simulink model "Non_Linear_Disturbance"  (R2024b)
settings: Solver=VariableStepAuto  StartTime=0.0  StopTime=500  RelTol=1e-9
settings Model: Creator=apm3  LastModifiedBy=baley

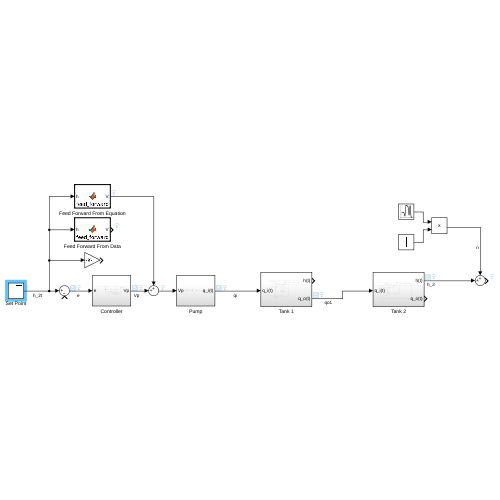
[thumbnail: Simulink's stored preview of the top-level diagram]
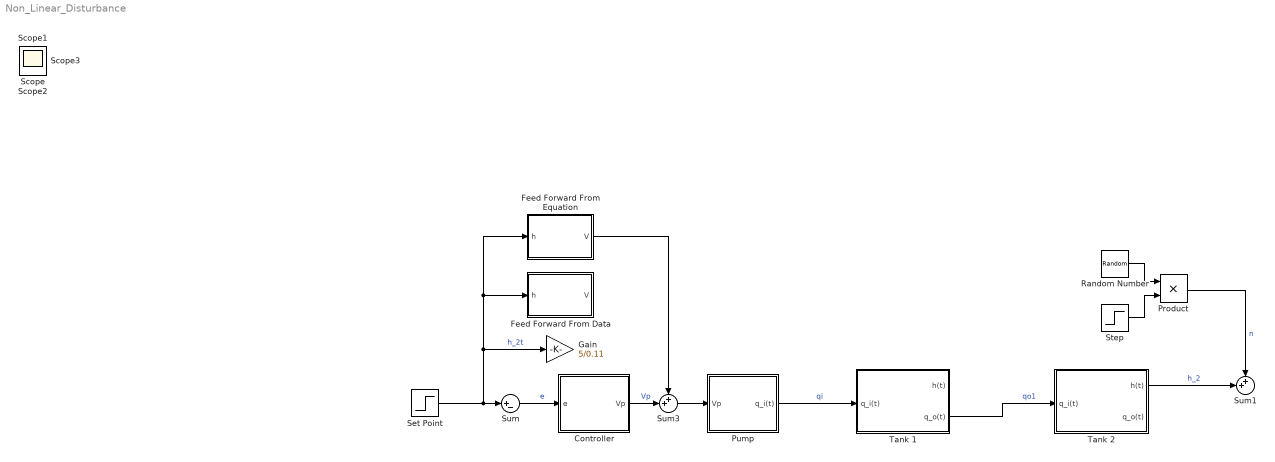
== system Non_Linear_Disturbance ==
  Controller : Subsystem
  Feed Forward From Data : MATLAB Function  TreatAsAtomicUnit=on
  Feed Forward From Equation : MATLAB Function  TreatAsAtomicUnit=on
  Gain : Gain  Gain=5/0.11
  Product : Product
  Pump : Subsystem
  Random Number : RandomNumber  Variance=0.000001  SampleTime=0.1
  Set Point : Step  After=0.2  SampleTime=0
  Step : Step  Time=1000  SampleTime=0
  Sum : Sum  Inputs=|+-
  Sum1 : Sum  Inputs=++|
  Sum3 : Sum  Inputs=++|
  Tank 1 : Subsystem
  Tank 2 : Subsystem
  Scope{,1..3} (4 alike) : Scope
  wires:
  Tank 1/2(q_o(t)) -> Tank 2/1(q_i(t))  "qo1"
  Pump/1(q_i(t)) -> Tank 1/1(q_i(t))  "qi"
  Sum/1 -> Controller/1(e)  "e"
  Set Point/1 -> Feed Forward From Equation/1(h), Feed Forward From Data/1(h), Gain/1, Sum/1  "h_2t"
  Tank 2/1(h(t)) -> Sum1/2  "h_2"
  Random Number/1 -> Product/1
  Step/1 -> Product/2
  Product/1 -> Sum1/1  "n"
  Controller/1(Vp) -> Sum3/2  "Vp"
  Sum3/1 -> Pump/1(Vp)
  Feed Forward From Equation/1(V) -> Sum3/1

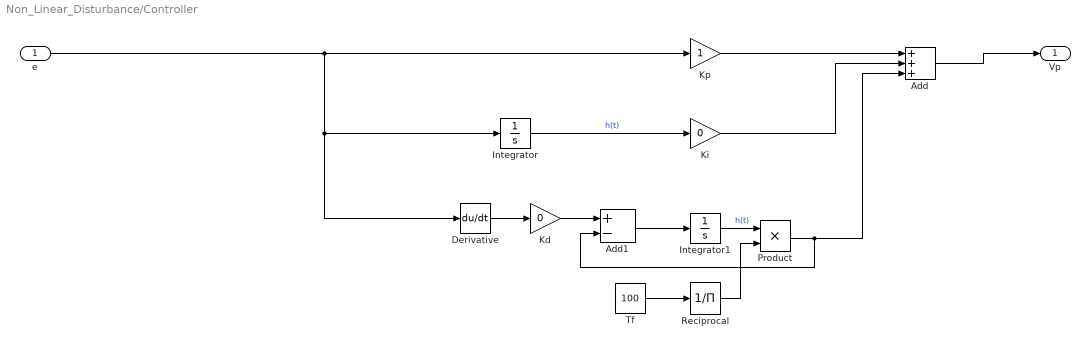
== system Non_Linear_Disturbance/Controller ==
  e : Inport
  Add : Sum  Inputs=+++
  Add1 : Sum  Inputs=+-
  Derivative : Derivative
  Integrator : Integrator
  Integrator1 : Integrator
  Kd : Gain  Gain=0
  Ki : Gain  Gain=0
  Kp : Gain
  Product : Product
  Reciprocal : Product  Inputs=/
  Tf : Constant  Value=100
  Vp : Outport
  wires:
  Kp/1 -> Add/1
  Add/1 -> Vp/1
  Ki/1 -> Add/2
  e/1 -> Derivative/1, Integrator/1, Kp/1
  Derivative/1 -> Kd/1
  Tf/1 -> Reciprocal/1
  Integrator/1 -> Ki/1  "h(t)"
  Kd/1 -> Add1/1
  Add1/1 -> Integrator1/1
  Integrator1/1 -> Product/1  "h(t)"
  Reciprocal/1 -> Product/2
  Product/1 -> Add1/2, Add/3

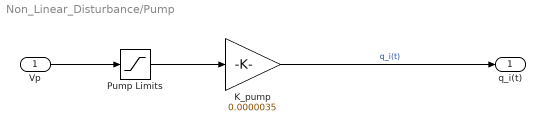
== system Non_Linear_Disturbance/Pump ==
  Vp : Inport
  K_pump : Gain  Gain=0.0000035
  Pump Limits : Saturate  UpperLimit=12  LowerLimit=0
  q_i(t) : Outport
  wires:
  K_pump/1 -> q_i(t)/1  "q_i(t)"
  Vp/1 -> Pump Limits/1
  Pump Limits/1 -> K_pump/1

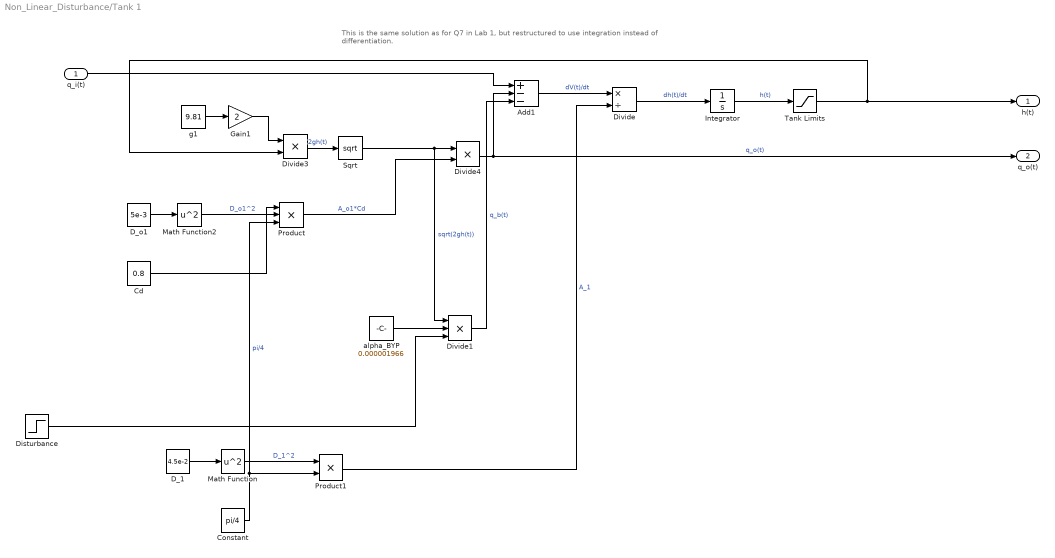
== system Non_Linear_Disturbance/Tank 1 ==
  note: This is the same solution as for Q7 in Lab 1, but restructured to use integration instead of differentiation.
  q_i(t) : Inport
  Add1 : Sum  Inputs=+--
  Cd : Constant  Value=0.8
  Constant : Constant  Value=pi/4
  D_1 : Constant  Value=4.5e-2
  D_o1 : Constant  Value=5e-3
  Disturbance : Step  Time=200  SampleTime=0
  Divide : Product  Inputs=*/
  Divide1 : Product  Inputs=***
  Divide3 : Product  Inputs=**
  Divide4 : Product  Inputs=**
  Gain1 : Gain  Gain=2
  Integrator : Integrator
  Math Function : Math  Operator=square
  Math Function2 : Math  Operator=square
  Product : Product  Inputs=3
  Product1 : Product
  Sqrt : Sqrt
  Tank Limits : Saturate  UpperLimit=0.25  LowerLimit=0
  alpha_BYP : Constant  Value=0.000001966
  g1 : Constant  Value=9.81
  h(t) : Outport
  q_o(t) : Outport  Port=2
  wires:
  Math Function/1 -> Product1/1  "D_1^2"
  Cd/1 -> Product/1
  D_o1/1 -> Math Function2/1
  Product1/1 -> Divide/2  "A_1"
  Constant/1 -> Product1/2, Product/3  "pi/4"
  D_1/1 -> Math Function/1
  Product/1 -> Divide4/2  "A_o1*Cd"
  Math Function2/1 -> Product/2  "D_o1^2"
  Divide3/1 -> Sqrt/1  "2gh(t)"
  Gain1/1 -> Divide3/1
  g1/1 -> Gain1/1
  Sqrt/1 -> Divide1/1, Divide4/1  "sqrt(2gh(t))"
  q_i(t)/1 -> Add1/1
  Divide4/1 -> q_o(t)/1, Add1/2  "q_o(t)"
  Add1/1 -> Divide/1  "dV(t)/dt"
  Divide/1 -> Integrator/1  "dh(t)/dt"
  Integrator/1 -> Tank Limits/1  "h(t)"
  Tank Limits/1 -> Divide3/2, h(t)/1
  Divide1/1 -> Add1/3  "q_b(t)"
  Disturbance/1 -> Divide1/3
  alpha_BYP/1 -> Divide1/2

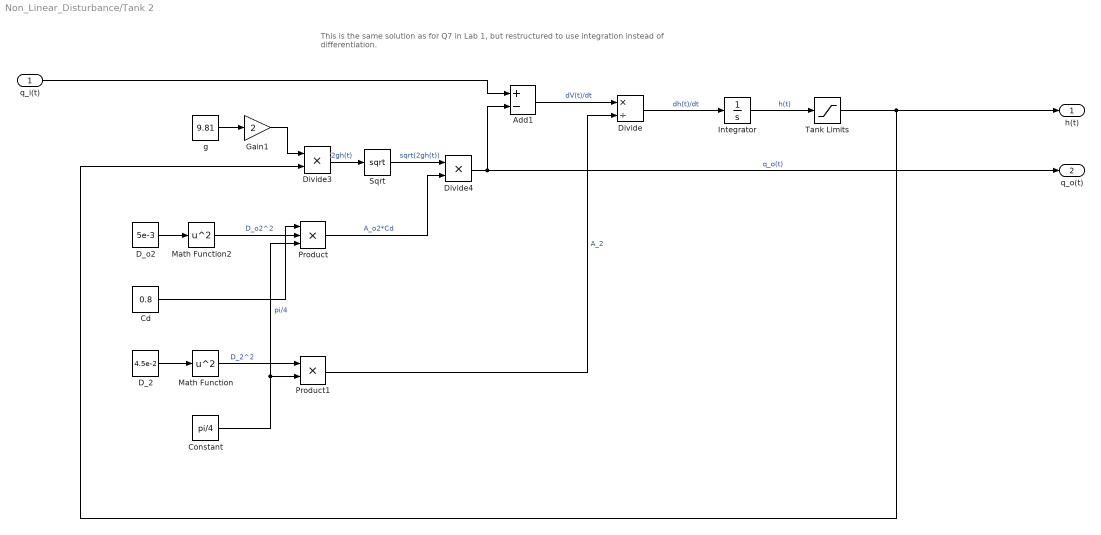
== system Non_Linear_Disturbance/Tank 2 ==
  note: This is the same solution as for Q7 in Lab 1, but restructured to use integration instead of differentiation.
  q_i(t) : Inport
  Add1 : Sum  Inputs=+-
  Cd : Constant  Value=0.8
  Constant : Constant  Value=pi/4
  D_2 : Constant  Value=4.5e-2
  D_o2 : Constant  Value=5e-3
  Divide : Product  Inputs=*/
  Divide3 : Product  Inputs=**
  Divide4 : Product  Inputs=**
  Gain1 : Gain  Gain=2
  Integrator : Integrator
  Math Function : Math  Operator=square
  Math Function2 : Math  Operator=square
  Product : Product  Inputs=3
  Product1 : Product
  Sqrt : Sqrt
  Tank Limits : Saturate  UpperLimit=0.25  LowerLimit=0
  g : Constant  Value=9.81
  h(t) : Outport
  q_o(t) : Outport  Port=2
  wires:
  Math Function/1 -> Product1/1  "D_2^2"
  Cd/1 -> Product/1
  D_o2/1 -> Math Function2/1
  Product1/1 -> Divide/2  "A_2"
  Constant/1 -> Product/3, Product1/2  "pi/4"
  D_2/1 -> Math Function/1
  Product/1 -> Divide4/2  "A_o2*Cd"
  Math Function2/1 -> Product/2  "D_o2^2"
  Divide3/1 -> Sqrt/1  "2gh(t)"
  Gain1/1 -> Divide3/1
  g/1 -> Gain1/1
  Sqrt/1 -> Divide4/1  "sqrt(2gh(t))"
  q_i(t)/1 -> Add1/1
  Divide4/1 -> q_o(t)/1, Add1/2  "q_o(t)"
  Add1/1 -> Divide/1  "dV(t)/dt"
  Divide/1 -> Integrator/1  "dh(t)/dt"
  Integrator/1 -> Tank Limits/1  "h(t)"
  Tank Limits/1 -> Divide3/2, h(t)/1

== matlab function Non_Linear_Disturbance/Feed Forward From Data ==
  data: h input; V output
function V = feed_forward(h)
    if h <= 0.063
        V = 79.37*h;
    elseif h <= 0.124
        V = 32.79*h + 2.937;
    else
        V = 26.32*h + 3.73;
    end

== matlab function Non_Linear_Disturbance/Feed Forward From Equation ==
  data: h input; V output
function V = feed_forward(h)
    V = 19.87*sqrt(h);
